simulink model "filtrationwhat"  (R2024a)
settings: Solver=VariableStepAuto  StartTime=0.0  StopTime=100000  RelTol=1e-3
libraries: dspfdesign x2, dspstat3 x1
settings Model: Creator=Lisa  LastModifiedBy=pupkinzalupkin
settings DataIOCC: Decimation=100
settings OptimizationCC: ReuseModelBlockBuffer=off
settings RTWCC: GPUComputeCapability=3.5

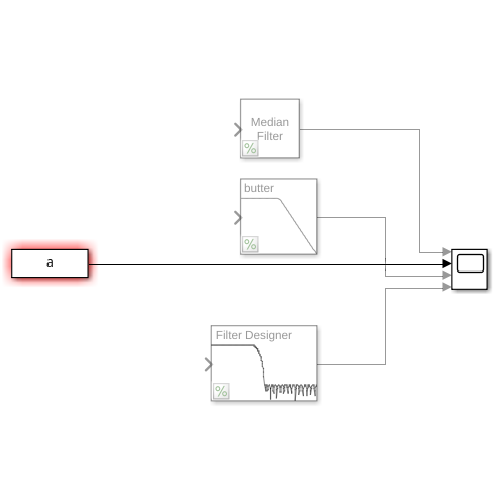
[thumbnail: Simulink's stored preview of the top-level diagram]
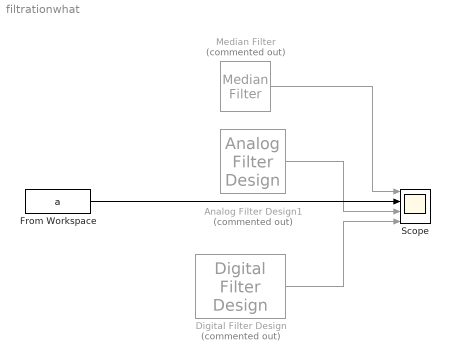
== system filtrationwhat ==
  Analog Filter Design1 : dspfdesign/Analog Filter Design  Commented=on  method=Butterworth  filttype=Lowpass  N=8  Wlo=30  Whi=80  Rp=2  Rs=40
  Digital Filter Design : dspfdesign/Digital Filter Design  Commented=on  mwdsp_browser_bugfix_var=off
  From Workspace : FromWorkspace  VariableName=a
  Median Filter : dspstat3/Median Filter  Commented=on  WindowLength=10  SimulateUsing=Code generation
  Scope : Scope  NumInputPorts=4
  wires:
  Analog Filter Design1/1 -> Scope/3
  Digital Filter Design/1 -> Scope/4
  Median Filter/1 -> Scope/1
  From Workspace/1 -> Scope/2
